simulink model "multidrug2022simulation"  (R2022b)
settings: Solver=FixedStepAuto  StartTime=0.0  StopTime=100  FixedStep=0.1  RelTol=1e-3
undefined symbols (not defined in the file): alpha1, alpha2, an, beta1, bn, DiscIntNeverNeededParam, gamma, k1, k2, k3, k4, lambda1, lambda2, r1, r2, r3, r4, T_star, tau1, tau2, tau23, tau32
libraries: slpidlib x2
settings Model: Creator=emirkenar  LastModifiedBy=kaganakar
settings SolverCC: AlgebraicLoopSolver=TrustRegion
settings DebuggingCC: UnconnectedInputMsg=warning  UnconnectedOutputMsg=warning  UnconnectedLineMsg=warning  SFMachineParentedDataDiag=warning  UnderSpecifiedDimensionMsg=warning
settings ModelReferenceCC: EnableRefExpFcnMdlSchedulingChecks=on
settings SFSimCC: CustomCodeUndefinedFunction=UseInterfaceOnly

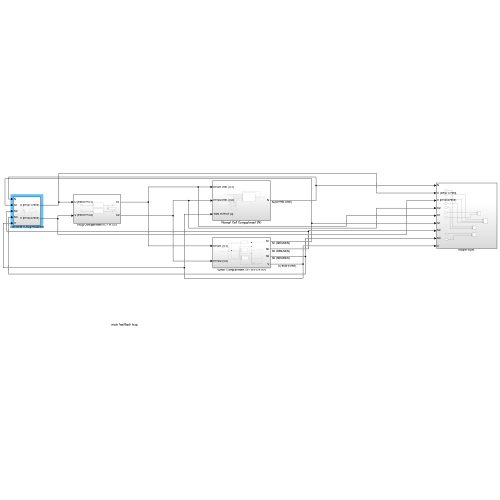
[thumbnail: Simulink's stored preview of the top-level diagram]
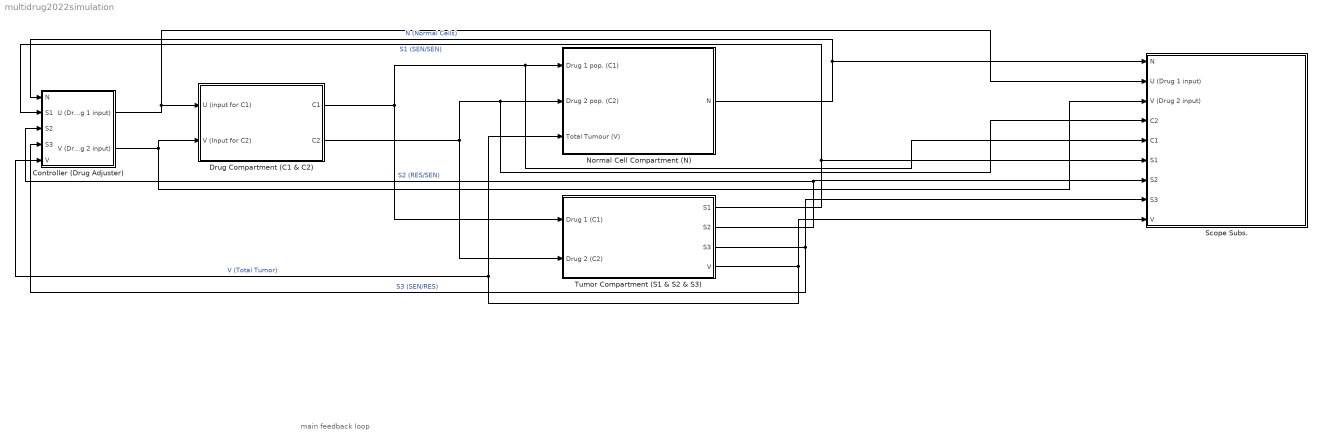
== system multidrug2022simulation ==
  note: main feedback loop
  Controller (Drug Adjuster) : Subsystem
  "Drug Compartment (C1 & C2) " : Subsystem
  Normal Cell Compartment (N) : Subsystem
  Scope Subs. : Subsystem
  Tumor Compartment (S1 & S2 & S3) : Subsystem
  wires:
  Controller (Drug Adjuster)/1(U (Drug 1 input)) -> Scope Subs./2(U (Drug 1 input)), "Drug Compartment (C1 & C2) "/1(U (input for C1))
  Controller (Drug Adjuster)/2(V (Drug 2 input)) -> "Drug Compartment (C1 & C2) "/2(V (Input for C2)), Scope Subs./3(V (Drug 2 input))
  "Drug Compartment (C1 & C2) "/1(C1) -> Tumor Compartment (S1 & S2 & S3)/1(Drug 1 (C1)), Scope Subs./5(C1), Normal Cell Compartment (N)/1(Drug 1 pop. (C1))
  "Drug Compartment (C1 & C2) "/2(C2) -> Tumor Compartment (S1 & S2 & S3)/2(Drug 2 (C2)), Scope Subs./4(C2), Normal Cell Compartment (N)/2(Drug 2 pop. (C2))
  Tumor Compartment (S1 & S2 & S3)/4(V) -> Normal Cell Compartment (N)/3(Total Tumour (V)), Controller (Drug Adjuster)/5(V), Scope Subs./9(V)  "V (Total Tumor)"
  Normal Cell Compartment (N)/1(N) -> Controller (Drug Adjuster)/1(N), Scope Subs./1(N)  "N (Normal Cells)"
  Tumor Compartment (S1 & S2 & S3)/1(S1) -> Scope Subs./6(S1), Controller (Drug Adjuster)/2(S1)  "S1 (SEN/SEN)"
  Tumor Compartment (S1 & S2 & S3)/2(S2) -> Controller (Drug Adjuster)/3(S2), Scope Subs./7(S2)  "S2 (RES/SEN)"
  Tumor Compartment (S1 & S2 & S3)/3(S3) -> Controller (Drug Adjuster)/4(S3), Scope Subs./8(S3)  "S3 (SEN/RES)"

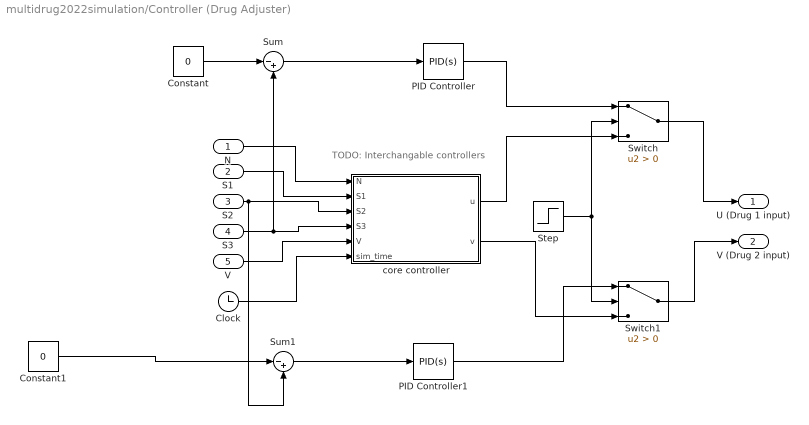
== system multidrug2022simulation/Controller (Drug Adjuster) ==
  note: TODO: Interchangable controllers
  N : Inport
  S1 : Inport  Port=2
  S2 : Inport  Port=3
  S3 : Inport  Port=4
  V : Inport  Port=5
  Clock : Clock
  Constant : Constant  Value=0
  Constant1 : Constant  Value=0
  PID Controller : slpidlib/PID Controller  Controller=PID  Form=Parallel  TimeDomain=Continuous-time  UseExternalTs=off  SampleTime=1  IntegratorMethod=Forward Euler  FilterMethod=Forward Euler  ControllerParametersSource=internal  P=10^-5  I=10^-7  UseKiTs=off  D=0  N=100  UseFilter=on  TunerSelectOption=Transfer Function Based (PID Tuner App)  InitialConditionSource=internal  InitialConditionForIntegrator=0  InitialConditionForFilter=0  DifferentiatorICPrevScaledInput=0  ExternalReset=none  TrackingMode=off  Kt=1  LimitOutput=off  SatLimitsSource=internal  UpperSaturationLimit=inf  LowerSaturationLimit=-inf  LinearizeAsGain=on  AntiWindupMode=none  Kb=1  LimitIntegrator=off  UpperIntegratorSaturationLimit=inf  LowerIntegratorSaturationLimit=-inf  POutMin=[]  POutMax=[]  IOutMin=[]  IOutMax=[]  DOutMin=[]  DOutMax=[]  NOutMin=[]  NOutMax=[]  SumOutMin=[]  SumOutMax=[]  SaturationOutMin=[]  SaturationOutMax=[]  PParamMin=[]  PParamMax=[]  IParamMin=[]  IParamMax=[]  DParamMin=[]  DParamMax=[]  NParamMin=[]  NParamMax=[]  KbParamMin=[]  KbParamMax=[]  KtParamMin=[]  KtParamMax=[]  KbOutMin=[]  KbOutMax=[]  KtOutMin=[]  KtOutMax=[]  IntegratorOutMin=[]  IntegratorOutMax=[]  FilterOutMin=[]  FilterOutMax=[]  SumI1OutMin=[]  SumI1OutMax=[]  SumI2OutMin=[]  SumI2OutMax=[]  SumI3OutMin=[]  SumI3OutMax=[]  SumI4OutMin=[]  SumI4OutMax=[]  SumDOutMin=[]  SumDOutMax=[]  DifferentiatorOutMin=[]  DifferentiatorOutMax=[]  FilterDiffOutCoefMin=[]  FilterDiffOutCoefMax=[]  ReciprocalOutMin=[]  ReciprocalOutMax=[]  SumDenOutMin=[]  SumDenOutMax=[]  SumNumOutMin=[]  SumNumOutMax=[]  DivideOutMin=[]  DivideOutMax=[]  UdiffTsProdOutMin=[]  UdiffTsProdOutMax=[]  NTsProdOutMin=[]  NTsProdOutMax=[]  UintegralTsProdOutMin=[]  UintegralTsProdOutMax=[]  UngainTsProdOutMin=[]  UngainTsProdOutMax=[]  ClampingZeroOutDataTypeStr=Inherit: Inherit via back propagation  ClampingZeroOutMin=[]  ClampingZeroOutMax=[]  FilterDenConstantOutDataTypeStr=Inherit: Inherit via back propagation  FilterDenConstantOutMin=[]  FilterDenConstantOutMax=[]  PCopyOutDataTypeStr=Inherit: Inherit via back propagation  PCopyOutMin=[]  PCopyOutMax=[]  NCopyOutDataTypeStr=Inherit: Inherit via back propagation  NCopyOutMin=[]  NCopyOutMax=[]  IntegratorContinuousStateAttributes=''  IntegratorStateMustResolveToSignalObject=off  IntegratorRTWStateStorageClass=Auto  FilterContinuousStateAttributes=''  FilterStateMustResolveToSignalObject=off  FilterRTWStateStorageClass=Auto  ParallelPVariant=InternalParameters  IdealPVariant=Disabled  IVariant=InternalParameters  DVariant=InternalParameters  IntegratorVariant=Continuous  SatVariant=Disabled  AWVariant=Passthrough  PCopyVariant=Disabled  TRVariant=Disabled  FdbkBlocksVariant=Forward  IdealPFdbkVariant=Disabled  SatFdbkVariant=Disabled  DerivativeFilterVariant=ContFilter  NVariant=InternalParameters  NCopyVariant=Disabled  FilterICVariant=InternalICsFilter  IntegratorICVariant=InternalICs  ExternalResetVariant=Disabled  TRSumVariant=Passthrough  SumFdbkVariant=Disabled  SumVariant=Sum_PID  TsampFilterVariant=InternalTs  TsampNgainVariant=Passthrough  TsampIntegralVariant=Passthrough  ExternalSaturationOutDataTypeStr=Inherit: Same as second input
  PID Controller1 : slpidlib/PID Controller  Controller=PID  Form=Parallel  TimeDomain=Continuous-time  UseExternalTs=off  SampleTime=1  IntegratorMethod=Forward Euler  FilterMethod=Forward Euler  ControllerParametersSource=internal  P=10^-5  I=10^-7  UseKiTs=off  D=0  N=100  UseFilter=on  TunerSelectOption=Transfer Function Based (PID Tuner App)  InitialConditionSource=internal  InitialConditionForIntegrator=0  InitialConditionForFilter=0  DifferentiatorICPrevScaledInput=0  ExternalReset=none  TrackingMode=off  Kt=1  LimitOutput=off  SatLimitsSource=internal  UpperSaturationLimit=inf  LowerSaturationLimit=-inf  LinearizeAsGain=on  AntiWindupMode=none  Kb=1  LimitIntegrator=off  UpperIntegratorSaturationLimit=inf  LowerIntegratorSaturationLimit=-inf  POutMin=[]  POutMax=[]  IOutMin=[]  IOutMax=[]  DOutMin=[]  DOutMax=[]  NOutMin=[]  NOutMax=[]  SumOutMin=[]  SumOutMax=[]  SaturationOutMin=[]  SaturationOutMax=[]  PParamMin=[]  PParamMax=[]  IParamMin=[]  IParamMax=[]  DParamMin=[]  DParamMax=[]  NParamMin=[]  NParamMax=[]  KbParamMin=[]  KbParamMax=[]  KtParamMin=[]  KtParamMax=[]  KbOutMin=[]  KbOutMax=[]  KtOutMin=[]  KtOutMax=[]  IntegratorOutMin=[]  IntegratorOutMax=[]  FilterOutMin=[]  FilterOutMax=[]  SumI1OutMin=[]  SumI1OutMax=[]  SumI2OutMin=[]  SumI2OutMax=[]  SumI3OutMin=[]  SumI3OutMax=[]  SumI4OutMin=[]  SumI4OutMax=[]  SumDOutMin=[]  SumDOutMax=[]  DifferentiatorOutMin=[]  DifferentiatorOutMax=[]  FilterDiffOutCoefMin=[]  FilterDiffOutCoefMax=[]  ReciprocalOutMin=[]  ReciprocalOutMax=[]  SumDenOutMin=[]  SumDenOutMax=[]  SumNumOutMin=[]  SumNumOutMax=[]  DivideOutMin=[]  DivideOutMax=[]  UdiffTsProdOutMin=[]  UdiffTsProdOutMax=[]  NTsProdOutMin=[]  NTsProdOutMax=[]  UintegralTsProdOutMin=[]  UintegralTsProdOutMax=[]  UngainTsProdOutMin=[]  UngainTsProdOutMax=[]  ClampingZeroOutDataTypeStr=Inherit: Inherit via back propagation  ClampingZeroOutMin=[]  ClampingZeroOutMax=[]  FilterDenConstantOutDataTypeStr=Inherit: Inherit via back propagation  FilterDenConstantOutMin=[]  FilterDenConstantOutMax=[]  PCopyOutDataTypeStr=Inherit: Inherit via back propagation  PCopyOutMin=[]  PCopyOutMax=[]  NCopyOutDataTypeStr=Inherit: Inherit via back propagation  NCopyOutMin=[]  NCopyOutMax=[]  IntegratorContinuousStateAttributes=''  IntegratorStateMustResolveToSignalObject=off  IntegratorRTWStateStorageClass=Auto  FilterContinuousStateAttributes=''  FilterStateMustResolveToSignalObject=off  FilterRTWStateStorageClass=Auto  ParallelPVariant=InternalParameters  IdealPVariant=Disabled  IVariant=InternalParameters  DVariant=InternalParameters  IntegratorVariant=Continuous  SatVariant=Disabled  AWVariant=Passthrough  PCopyVariant=Disabled  TRVariant=Disabled  FdbkBlocksVariant=Forward  IdealPFdbkVariant=Disabled  SatFdbkVariant=Disabled  DerivativeFilterVariant=ContFilter  NVariant=InternalParameters  NCopyVariant=Disabled  FilterICVariant=InternalICsFilter  IntegratorICVariant=InternalICs  ExternalResetVariant=Disabled  TRSumVariant=Passthrough  SumFdbkVariant=Disabled  SumVariant=Sum_PID  TsampFilterVariant=InternalTs  TsampNgainVariant=Passthrough  TsampIntegralVariant=Passthrough  ExternalSaturationOutDataTypeStr=Inherit: Same as second input
  Step : Step  SampleTime=0
  Sum : Sum  Inputs=|-+
  Sum1 : Sum  Inputs=|-+
  Switch : Switch  Criteria=u2 > Threshold  SaturateOnIntegerOverflow=off  InputSameDT=off
  Switch1 : Switch  Criteria=u2 > Threshold  SaturateOnIntegerOverflow=off  InputSameDT=off
  core controller : MATLAB Function  TreatAsAtomicUnit=on
  U (Drug 1 input) : Outport  VectorParamsAs1DForOutWhenUnconnected=off
  V (Drug 2 input) : Outport  Port=2  VectorParamsAs1DForOutWhenUnconnected=off
  wires:
  N/1 -> core controller/1(N)
  S1/1 -> core controller/2(S1)
  S2/1 -> Sum1/2, core controller/3(S2)
  S3/1 -> Sum/2, core controller/4(S3)
  V/1 -> core controller/5(V)
  Clock/1 -> core controller/6(sim_time)
  Constant/1 -> Sum/1
  Sum/1 -> PID Controller/1
  Sum1/1 -> PID Controller1/1
  Constant1/1 -> Sum1/1
  core controller/1(u) -> Switch/3
  PID Controller/1 -> Switch/1
  Step/1 -> Switch1/2, Switch/2
  Switch1/1 -> V (Drug 2 input)/1
  Switch/1 -> U (Drug 1 input)/1
  core controller/2(v) -> Switch1/3
  PID Controller1/1 -> Switch1/1

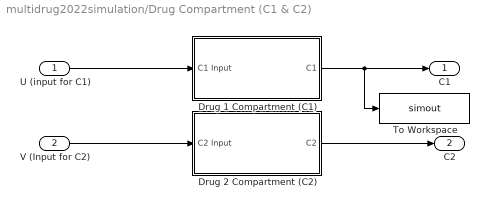
== system multidrug2022simulation/Drug Compartment (C1 & C2)  ==
  U (input for C1) : Inport
  V (Input for C2) : Inport  Port=2
  Drug 1 Compartment (C1) : Subsystem
  Drug 2 Compartment (C2) : Subsystem
  To Workspace : ToWorkspace  VariableName=simout  SaveFormat=Timeseries  SampleTime=-1
  C1 : Outport  VectorParamsAs1DForOutWhenUnconnected=off
  C2 : Outport  Port=2  VectorParamsAs1DForOutWhenUnconnected=off
  wires:
  U (input for C1)/1 -> Drug 1 Compartment (C1)/1(C1 Input)
  Drug 1 Compartment (C1)/1(C1) -> To Workspace/1, C1/1
  Drug 2 Compartment (C2)/1(C2) -> C2/1
  V (Input for C2)/1 -> Drug 2 Compartment (C2)/1("C2 Input ")

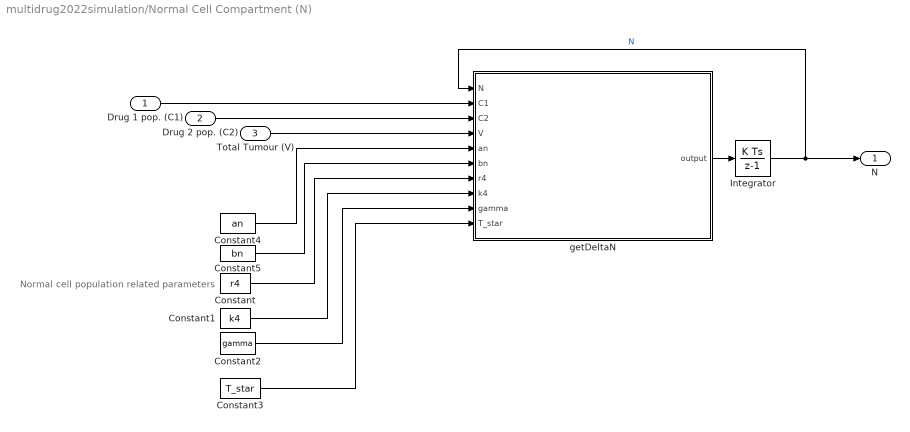
== system multidrug2022simulation/Normal Cell Compartment (N) ==
  note: Normal cell population related parameters
  Drug 1 pop. (C1) : Inport
  Drug 2 pop. (C2) : Inport  Port=2
  Total Tumour (V) : Inport  Port=3
  Constant : Constant  Value=r4
  Constant1 : Constant  Value=k4
  Constant2 : Constant  Value=gamma
  Constant3 : Constant  Value=T_star
  Constant4 : Constant  Value=an
  Constant5 : Constant  Value=bn
  Integrator : DiscreteIntegrator  InitialCondition=10*10^5  SampleTime=-1  ICPrevOutput=DiscIntNeverNeededParam  ICPrevScaledInput=DiscIntNeverNeededParam
  getDeltaN : MATLAB Function  TreatAsAtomicUnit=on
  N : Outport  VectorParamsAs1DForOutWhenUnconnected=off
  wires:
  Total Tumour (V)/1 -> getDeltaN/4(V)
  Drug 1 pop. (C1)/1 -> getDeltaN/2(C1)
  Drug 2 pop. (C2)/1 -> getDeltaN/3(C2)
  Constant5/1 -> getDeltaN/6(bn)
  Constant1/1 -> getDeltaN/8(k4)
  Constant4/1 -> getDeltaN/5(an)
  Constant/1 -> getDeltaN/7(r4)
  Integrator/1 -> N/1, getDeltaN/1(N)  "N"
  Constant3/1 -> getDeltaN/10(T_star)
  getDeltaN/1(output) -> Integrator/1
  Constant2/1 -> getDeltaN/9(gamma)

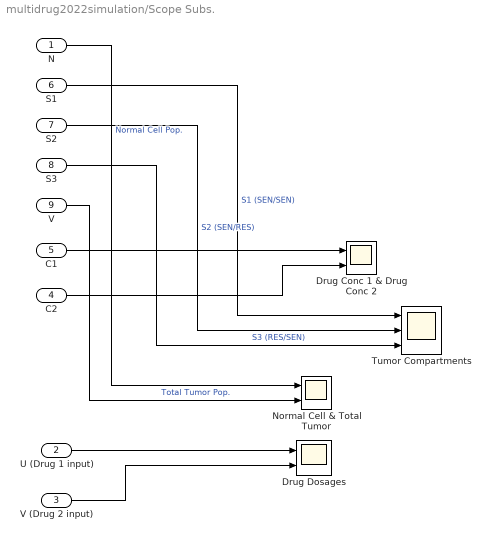
== system multidrug2022simulation/Scope Subs. ==
  N : Inport
  U (Drug 1 input) : Inport  Port=2
  V (Drug 2 input) : Inport  Port=3
  C2 : Inport  Port=4
  C1 : Inport  Port=5
  S1 : Inport  Port=6
  S2 : Inport  Port=7
  S3 : Inport  Port=8
  V : Inport  Port=9
  "Drug Conc 1 & Drug Conc 2 " : Scope  NumInputPorts=2
  Drug Dosages : Scope  NumInputPorts=2
  Normal Cell & Total Tumor : Scope  NumInputPorts=2
  Tumor Compartments : Scope  NumInputPorts=3
  wires:
  N/1 -> Normal Cell & Total Tumor/1  "Normal Cell Pop."
  V/1 -> Normal Cell & Total Tumor/2  "Total Tumor Pop."
  S1/1 -> Tumor Compartments/1  "S1 (SEN/SEN)"
  S2/1 -> Tumor Compartments/2  "S2 (SEN/RES)"
  S3/1 -> Tumor Compartments/3  "S3 (RES/SEN)"
  C1/1 -> "Drug Conc 1 & Drug Conc 2 "/1
  C2/1 -> "Drug Conc 1 & Drug Conc 2 "/2
  U (Drug 1 input)/1 -> Drug Dosages/1
  V (Drug 2 input)/1 -> Drug Dosages/2

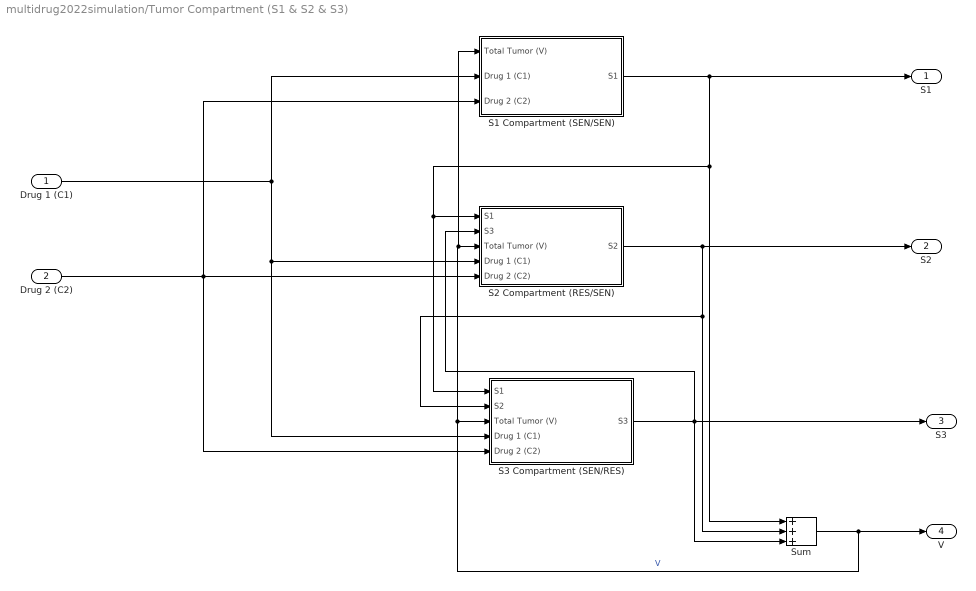
== system multidrug2022simulation/Tumor Compartment (S1 & S2 & S3) ==
  Drug 1 (C1) : Inport
  Drug 2 (C2) : Inport  Port=2
  S1 Compartment (SEN/SEN) : Subsystem
  S2 Compartment (RES/SEN) : Subsystem
  S3 Compartment (SEN/RES) : Subsystem
  Sum : Sum  Inputs=+++
  S1 : Outport  VectorParamsAs1DForOutWhenUnconnected=off
  S2 : Outport  Port=2  VectorParamsAs1DForOutWhenUnconnected=off
  S3 : Outport  Port=3  VectorParamsAs1DForOutWhenUnconnected=off
  V : Outport  Port=4  VectorParamsAs1DForOutWhenUnconnected=off
  wires:
  Sum/1 -> S1 Compartment (SEN/SEN)/1(Total Tumor (V)), S2 Compartment (RES/SEN)/3(Total Tumor (V)), S3 Compartment (SEN/RES)/3(Total Tumor (V)), V/1  "V"
  S2 Compartment (RES/SEN)/1(S2) -> S3 Compartment (SEN/RES)/2(S2), Sum/2, S2/1
  S3 Compartment (SEN/RES)/1(S3) -> S2 Compartment (RES/SEN)/2(S3), Sum/3, S3/1
  S1 Compartment (SEN/SEN)/1(S1) -> S3 Compartment (SEN/RES)/1(S1), S2 Compartment (RES/SEN)/1(S1), Sum/1, S1/1
  Drug 1 (C1)/1 -> S3 Compartment (SEN/RES)/4("Drug 1 (C1) "), S2 Compartment (RES/SEN)/4(Drug 1 (C1)), S1 Compartment (SEN/SEN)/2(Drug 1 (C1))
  Drug 2 (C2)/1 -> S3 Compartment (SEN/RES)/5(Drug 2 (C2)), S2 Compartment (RES/SEN)/5(Drug 2 (C2)), S1 Compartment (SEN/SEN)/3(Drug 2 (C2))

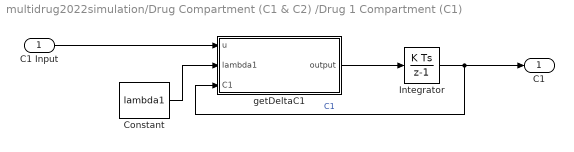
== system multidrug2022simulation/Drug Compartment (C1 & C2) /Drug 1 Compartment (C1) ==
  C1 Input : Inport
  Constant : Constant  Value=lambda1
  Integrator : DiscreteIntegrator  SampleTime=-1  ICPrevOutput=DiscIntNeverNeededParam  ICPrevScaledInput=DiscIntNeverNeededParam
  getDeltaC1 : MATLAB Function  TreatAsAtomicUnit=on
  C1 : Outport  VectorParamsAs1DForOutWhenUnconnected=off
  wires:
  C1 Input/1 -> getDeltaC1/1(u)
  Integrator/1 -> C1/1, getDeltaC1/3(C1)  "C1"
  getDeltaC1/1(output) -> Integrator/1
  Constant/1 -> getDeltaC1/2(lambda1)

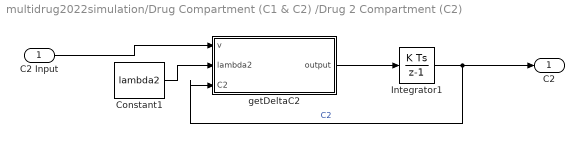
== system multidrug2022simulation/Drug Compartment (C1 & C2) /Drug 2 Compartment (C2) ==
  "C2 Input " : Inport
  Constant1 : Constant  Value=lambda2
  Integrator1 : DiscreteIntegrator  SampleTime=-1  ICPrevOutput=DiscIntNeverNeededParam  ICPrevScaledInput=DiscIntNeverNeededParam
  getDeltaC2 : MATLAB Function  TreatAsAtomicUnit=on
  C2 : Outport  VectorParamsAs1DForOutWhenUnconnected=off
  wires:
  "C2 Input "/1 -> getDeltaC2/1(v)
  getDeltaC2/1(output) -> Integrator1/1
  Integrator1/1 -> C2/1, getDeltaC2/3(C2)  "C2"
  Constant1/1 -> getDeltaC2/2(lambda2)

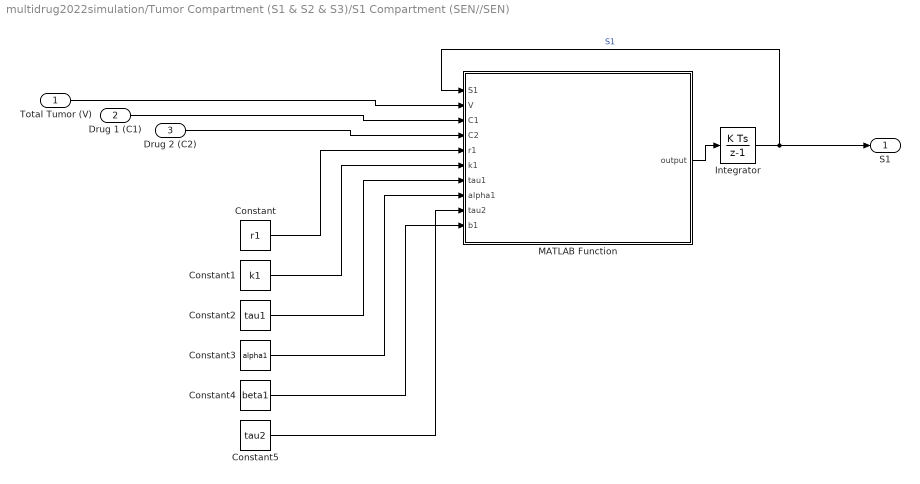
== system multidrug2022simulation/Tumor Compartment (S1 & S2 & S3)/S1 Compartment (SEN//SEN) ==
  Total Tumor (V) : Inport
  Drug 1 (C1) : Inport  Port=2
  Drug 2 (C2) : Inport  Port=3
  Constant : Constant  Value=r1
  Constant1 : Constant  Value=k1
  Constant2 : Constant  Value=tau1
  Constant3 : Constant  Value=alpha1
  Constant4 : Constant  Value=beta1
  Constant5 : Constant  Value=tau2
  Integrator : DiscreteIntegrator  InitialCondition=7*10^5  SampleTime=-1  ICPrevOutput=DiscIntNeverNeededParam  ICPrevScaledInput=DiscIntNeverNeededParam
  MATLAB Function : MATLAB Function  TreatAsAtomicUnit=on
  S1 : Outport  VectorParamsAs1DForOutWhenUnconnected=off
  wires:
  Constant2/1 -> MATLAB Function/7(tau1)
  Constant1/1 -> MATLAB Function/6(k1)
  Integrator/1 -> S1/1, MATLAB Function/1(S1)  "S1"
  Constant/1 -> MATLAB Function/5(r1)
  MATLAB Function/1(output) -> Integrator/1
  Constant3/1 -> MATLAB Function/8(alpha1)
  Constant4/1 -> MATLAB Function/10(b1)
  Total Tumor (V)/1 -> MATLAB Function/2(V)
  Drug 1 (C1)/1 -> MATLAB Function/3(C1)
  Drug 2 (C2)/1 -> MATLAB Function/4(C2)
  Constant5/1 -> MATLAB Function/9(tau2)

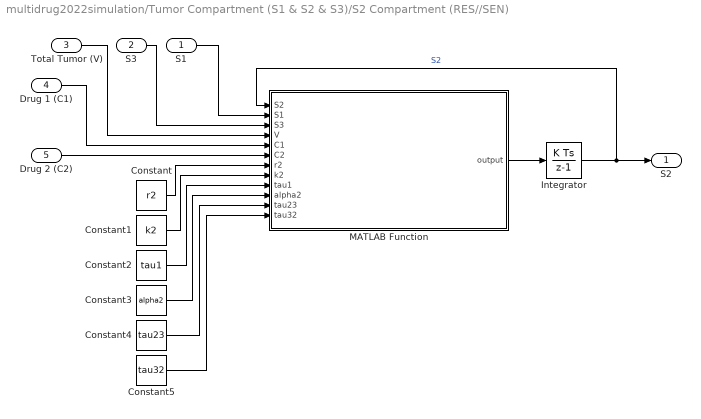
== system multidrug2022simulation/Tumor Compartment (S1 & S2 & S3)/S2 Compartment (RES//SEN) ==
  S1 : Inport
  S3 : Inport  Port=2
  Total Tumor (V) : Inport  Port=3
  Drug 1 (C1) : Inport  Port=4
  Drug 2 (C2) : Inport  Port=5
  Constant : Constant  Value=r2
  Constant1 : Constant  Value=k2
  Constant2 : Constant  Value=tau1
  Constant3 : Constant  Value=alpha2
  Constant4 : Constant  Value=tau23
  Constant5 : Constant  Value=tau32
  Integrator : DiscreteIntegrator  InitialCondition=10*10^4  SampleTime=-1  ICPrevOutput=DiscIntNeverNeededParam  ICPrevScaledInput=DiscIntNeverNeededParam
  MATLAB Function : MATLAB Function  TreatAsAtomicUnit=on
  S2 : Outport  VectorParamsAs1DForOutWhenUnconnected=off
  wires:
  Constant2/1 -> MATLAB Function/9(tau1)
  MATLAB Function/1(output) -> Integrator/1
  Constant5/1 -> MATLAB Function/12(tau32)
  Constant/1 -> MATLAB Function/7(r2)
  Constant4/1 -> MATLAB Function/11(tau23)
  Constant1/1 -> MATLAB Function/8(k2)
  Constant3/1 -> MATLAB Function/10(alpha2)
  Integrator/1 -> MATLAB Function/1(S2), S2/1  "S2"
  S1/1 -> MATLAB Function/2(S1)
  S3/1 -> MATLAB Function/3(S3)
  Total Tumor (V)/1 -> MATLAB Function/4(V)
  Drug 1 (C1)/1 -> MATLAB Function/5(C1)
  Drug 2 (C2)/1 -> MATLAB Function/6(C2)

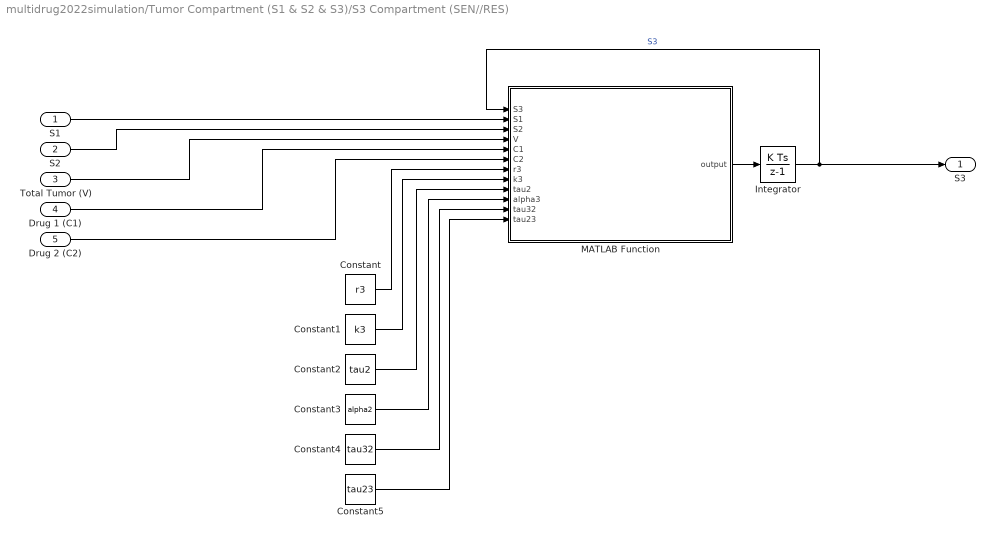
== system multidrug2022simulation/Tumor Compartment (S1 & S2 & S3)/S3 Compartment (SEN//RES) ==
  S1 : Inport
  S2 : Inport  Port=2
  Total Tumor (V) : Inport  Port=3
  "Drug 1 (C1) " : Inport  Port=4
  Drug 2 (C2) : Inport  Port=5
  Constant : Constant  Value=r3
  Constant1 : Constant  Value=k3
  Constant2 : Constant  Value=tau2
  Constant3 : Constant  Value=alpha2
  Constant4 : Constant  Value=tau32
  Constant5 : Constant  Value=tau23
  Integrator : DiscreteIntegrator  InitialCondition=10*10^4  SampleTime=-1  ICPrevOutput=DiscIntNeverNeededParam  ICPrevScaledInput=DiscIntNeverNeededParam
  MATLAB Function : MATLAB Function  TreatAsAtomicUnit=on
  S3 : Outport  VectorParamsAs1DForOutWhenUnconnected=off
  wires:
  Total Tumor (V)/1 -> MATLAB Function/4(V)
  S1/1 -> MATLAB Function/2(S1)
  Constant2/1 -> MATLAB Function/9(tau2)
  Constant4/1 -> MATLAB Function/11(tau32)
  Constant5/1 -> MATLAB Function/12(tau23)
  Constant/1 -> MATLAB Function/7(r3)
  Constant1/1 -> MATLAB Function/8(k3)
  S2/1 -> MATLAB Function/3(S2)
  Integrator/1 -> S3/1, MATLAB Function/1(S3)  "S3"
  Constant3/1 -> MATLAB Function/10(alpha3)
  "Drug 1 (C1) "/1 -> MATLAB Function/5(C1)
  Drug 2 (C2)/1 -> MATLAB Function/6(C2)
  MATLAB Function/1(output) -> Integrator/1

== matlab function multidrug2022simulation/Controller (Drug Adjuster)/core controller ==
  settings: updateMethod=DISCRETE
  data: N input; u output [0..1]; S1 input; S2 input; S3 input; V input; v output [0..1]; sim_time input

function [u, v] = coreController(N, S1, S2, S3, V, sim_time)
% %Trial section to figure out the proper lambda1, lambda2, gamma values 
    if sim_time < 100
        u = 1;
        v = 1;
    else 
        u = 0;
        v = 0;
    end
%S1 -> Sensitive to the both drugs
%S2 -> Sensitive to the only V
%S3 -> Sensitive to the only U


% The control section
%     persistent integralU;
%     persistent integralV;
%     persistent previousErrorU;
%     persistent previousErrorV;
%     if isempty(integralU)
%         integralU = 0;
%     end
%      if isempty(integralV)
%         integralV = 0;
%      end
%       if isempty(previousErrorU)
%         previousErrorU = 0;
%     end
% 
%     if isempty(previousErrorV)
%         previousErrorV = 0;
%     end
% 
%     comp2Tumor = S2;
%     comp3Tumor = S3;
%     targetValue = 0;
%     errorU = comp3Tumor - targetValue;
%     KpU = 10^-6;
%     KiU = 10^-8;
%     KdU = 0;
%     proportionalU = KpU*errorU;
%     integralU = integralU + KiU*errorU;
%     derivativeU = KdU*(errorU-previousErrorU)
%     signalU = proportionalU + integralU + derivativeU
%     u = signalU;
%      
%     errorV = comp2Tumor - targetValue;
% 
%     KpV = 10^-6;
%     KiV = 10^-8;
%     KdV = 0;
%     proportionalV = KpV*errorV
%     integralV = integralV + KiV*errorV;
%     derivativeV = KdV*(errorV-previousErrorV);
%     signalV = proportionalV + integralV + derivativeV;
%     v = signalV
% 
%     %v = Kp*error
%     if u > 0.5
%         u = 1
%     else
%         u = 0
%     end
%     if v > 0.5
%         v = 1
%     else
%         v = 0
%     end


end

== matlab function multidrug2022simulation/Drug Compartment (C1 & C2) /Drug 1 Compartment (C1)/getDeltaC1 ==
  data: u input; output output; lambda1 input; C1 input
function output = getDeltaC1(u,lambda1,C1)
    output = u- lambda1*C1;
end

== matlab function multidrug2022simulation/Drug Compartment (C1 & C2) /Drug 2 Compartment (C2)/getDeltaC2 ==
  data: v input; output output; lambda2 input; C2 input
function output = getDeltaC2(v,lambda2,C2)
    output = v-lambda2*C2;
end

== matlab function multidrug2022simulation/Normal Cell Compartment (N)/getDeltaN ==
  data: N input; C1 input; C2 input; V input; an input; bn input; r4 input; output output; k4 input; gamma input; T_star input
function output = getDeltaN(N,C1,C2,V,an,bn,r4,k4,gamma,T_star)
    output = r4*N*(1-N/k4)+gamma*V*(1-V/T_star)-an*(1-exp(-C1))*N-bn*(1-exp(-C2))*N;
end

== matlab function multidrug2022simulation/Tumor Compartment (S1 & S2 & S3)/S1 Compartment (SEN//SEN)/MATLAB Function ==
  data: S1 input; V input; C1 input; C2 input; r1 input; output output; k1 input; tau1 input; alpha1 input; tau2 input; b1 input
function output = getDeltaS1(S1,V,C1,C2,r1,k1,tau1,alpha1,tau2, b1)
    output = r1*S1*(1-(V)/(k1))-tau1*S1 - alpha1*(1-exp(-C1))*S1-b1*(1-exp(-C2))*S1 - tau2*S1;
    
end

== matlab function multidrug2022simulation/Tumor Compartment (S1 & S2 & S3)/S2 Compartment (RES//SEN)/MATLAB Function ==
  data: S2 input; S1 input; S3 input; V input; C1 input; C2 input; r2 input; output output; k2 input; tau1 input; alpha2 input; tau23 input; tau32 input
function output = getDeltaS2(S2,S1,S3,V,C1,C2,r2,k2,tau1,alpha2,tau23,tau32)
    output = r2*S2*(1-(V)/(k2))+tau1*S1-alpha2*(1-exp(-C2))*S2 -tau23*(1-exp(-C2))*S2+tau32*(1-exp(-C1)*S3);
    
end

== matlab function multidrug2022simulation/Tumor Compartment (S1 & S2 & S3)/S3 Compartment (SEN//RES)/MATLAB Function ==
  data: S3 input; S1 input; S2 input; V input; C1 input; C2 input; r3 input; output output; k3 input; tau2 input; alpha3 input; tau32 input; tau23 input
function output = getDeltaS3(S3,S1,S2,V,C1,C2,r3,k3,tau2,alpha3,tau32,tau23)
    output = r3*S3*(1-V/k3)+tau2*S1-alpha3*(1-exp(-C1))*S3 - tau32*(1-exp(-C1))*S3 + tau23*(1-exp(-C2))*S2;
end
